simulink model "chap14_1sim"  (Simulink 7.7)
settings: Solver=ode45  StartTime=0.0  StopTime=10  FixedStep=0.001  RelTol=1e-3
settings Model: Creator=ljk  LastModifiedBy=ljk  ExtModeTrigMode=oneshot  ExtModeArmWhenConnect=off
settings DataIOCC: LimitDataPoints=off  SignalLoggingName=sigsOut
settings OptimizationCC: BooleanDataType=off
settings DebuggingCC: SaveWithParameterizedLinksMsg=none  SignalResolutionControl=TryResolveAllWithWarning  SolverPrmCheckMsg=none  MultiTaskDSMMsg=warning  MultiTaskCondExecSysMsg=none  StrictBusMsg=None
settings HardwareCC: TargetUnknown=on
settings RTWCC: IncludeERTFirstTime=on

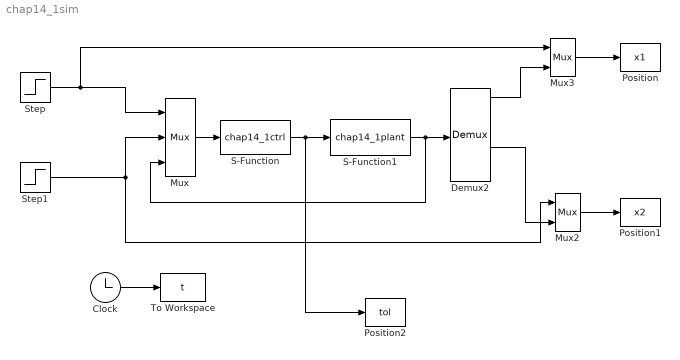
== system chap14_1sim ==
  Clock : Clock
      settings: Decimation=10
  Demux2 : Demux
  Mux : Mux  Inputs=3
  Mux2 : Mux  Inputs=2
  Mux3 : Mux  Inputs=2
  Position : ToWorkspace  VariableName=x1  SampleTime=-1  SaveFormat=Array
  Position1 : ToWorkspace  VariableName=x2  SampleTime=-1  SaveFormat=Array
  Position2 : ToWorkspace  VariableName=tol  SampleTime=-1  SaveFormat=Array
  S-Function : S-Function  FunctionName=chap14_1ctrl  EnableBusSupport=off
  S-Function1 : S-Function  FunctionName=chap14_1plant  EnableBusSupport=off
  Step : Step  Time=0  SampleTime=0
  Step1 : Step  Time=0  SampleTime=0
  To Workspace : ToWorkspace  VariableName=t  SampleTime=-1  SaveFormat=Array
  wires:
  Mux/1 -> S-Function/1
  Mux2/1 -> Position1/1
  Step/1 -> Mux/1, Mux3/1
  Mux3/1 -> Position/1
  S-Function/1 -> S-Function1/1, Position2/1
  Step1/1 -> Mux/2, Mux2/1
  Demux2/1 -> Mux3/2
  S-Function1/1 -> Demux2/1, Mux/3
  Clock/1 -> To Workspace/1
  Demux2/3 -> Mux2/2
